simulink model "Simulink"  (R2020b)
settings: Solver=ode45  StartTime=0.0  StopTime=1  RelTol=1e-6  AbsTol=1e-6
values from neighbouring files (symbols this model uses):
  A = 136    [Main.m]
  B = 0    [Main.m]
  iab_0 = [ia_0;ib_0]    [Main.m]
  Jm = 0.00027    [Main.m]
  L = 0.03    [Main.m]
  lamda_m = 0.3200    (= 0.32)    [Main.m]
  np = 5    [Main.m]
  omega_0 = 0    [Main.m]
  R = 6.25    [Main.m]
  theta_0 = 0    [Main.m]
  TL1 = 0.151    [Main.m]
  W = 74    [Main.m]
settings Model: Creator=sokra  LastModifiedBy=sokra
settings SolverCC: AutoScaleAbsTol=off

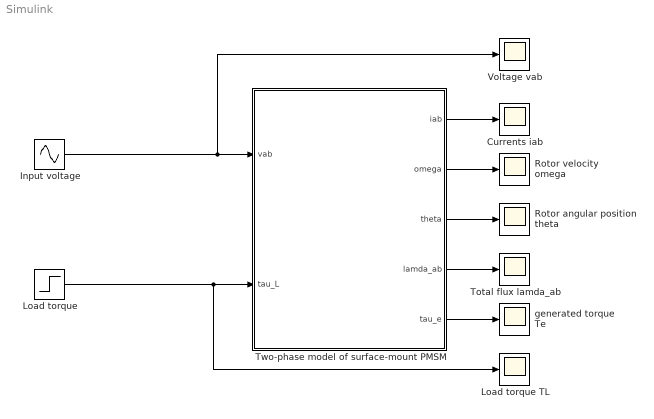
== system Simulink ==
  Currents iab : Scope
  Input voltage : Sin  Amplitude=A  Frequency=W  Phase=[pi/2;0]  SampleTime=0
  Load torque : Step  Time=0.5  After=TL1  SampleTime=0
  Load torque TL : Scope
  Rotor angular position theta : Scope
  "Rotor velocity omega " : Scope
  Total flux lamda_ab : Scope
  Two-phase model of surface-mount PMSM : Subsystem
  Voltage vab : Scope
  generated torque Te : Scope
  wires:
  Two-phase model of surface-mount PMSM/1(iab) -> Currents iab/1
  Two-phase model of surface-mount PMSM/2(omega) -> "Rotor velocity omega "/1
  Two-phase model of surface-mount PMSM/5(tau_e) -> generated torque Te/1
  Two-phase model of surface-mount PMSM/3(theta) -> Rotor angular position theta/1
  Two-phase model of surface-mount PMSM/4(lamda_ab) -> Total flux lamda_ab/1
  Load torque/1 -> Load torque TL/1, Two-phase model of surface-mount PMSM/2(tau_L)
  Input voltage/1 -> Voltage vab/1, Two-phase model of surface-mount PMSM/1(vab)

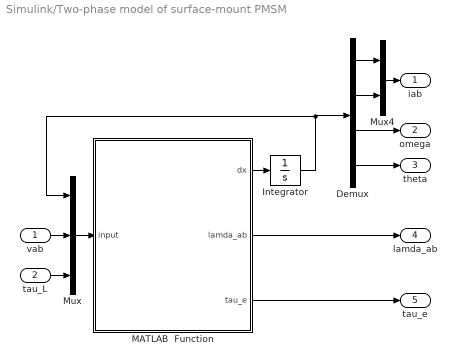
== system Simulink/Two-phase model of surface-mount PMSM ==
  vab : Inport
  tau_L : Inport  Port=2
  Demux : Demux
  Integrator : Integrator  InitialCondition=[iab_0;omega_0;theta_0]
  MATLAB  Function : MATLAB Function  TreatAsAtomicUnit=on
  Mux : Mux  Inputs=3
  Mux4 : Mux  Inputs=2
  iab : Outport
  omega : Outport  Port=2
  theta : Outport  Port=3
  lamda_ab : Outport  Port=4
  tau_e : Outport  Port=5
  wires:
  Mux4/1 -> iab/1
  MATLAB  Function/1(dx) -> Integrator/1
  Mux/1 -> MATLAB  Function/1(input)
  Integrator/1 -> Demux/1, Mux/1
  Demux/2 -> Mux4/2
  vab/1 -> Mux/2
  MATLAB  Function/2(lamda_ab) -> lamda_ab/1
  Demux/1 -> Mux4/1
  tau_L/1 -> Mux/3
  Demux/3 -> omega/1
  Demux/4 -> theta/1
  MATLAB  Function/3(tau_e) -> tau_e/1

== matlab function Simulink/Two-phase model of surface-mount PMSM/MATLAB  Function ==
  data: input input; dx output; lamda_ab output; R parameter; L parameter; lamda_m parameter; np parameter; Jm parameter; B parameter; tau_e output
function [dx,lamda_ab,tau_e]  = fcn(input,R, L, lamda_m, np, Jm, B)
ia=input(1);
ib=input(2);
iab=[ia;ib];
omega=input(3);
theta=input(4);
va=input(5);
vb=input(6);
vab=[va;vb];
tau_L=input(7);

%%%%%%%
C=[cos(np*theta);sin(np*theta)];
J=[0 -1;1 0];
dC=np*J*C;
%%%%%%%
dot_iab=(1/L)*(-R*iab-omega*lamda_m*dC+vab);
dot_omega=(1/Jm)*(-B*omega+lamda_m*iab'*dC-tau_L);
dot_theta=omega;
lamda_ab=L*iab+lamda_m*C;
dx = [dot_iab;dot_omega;dot_theta];
tau_e = np * iab' * J * lamda_ab;
end
